simulink model "sampleModel1852"  (R2023a)
settings: Solver=VariableStepAuto  StartTime=0.0  StopTime=10.0  RelTol=1e-3
libraries: hdlsllib x3, simulink x2
settings Model: Creator=user1  LastModifiedBy=user1

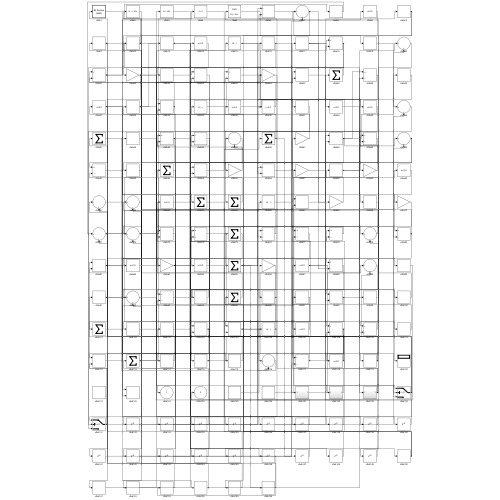
[thumbnail: Simulink's stored preview of the top-level diagram]
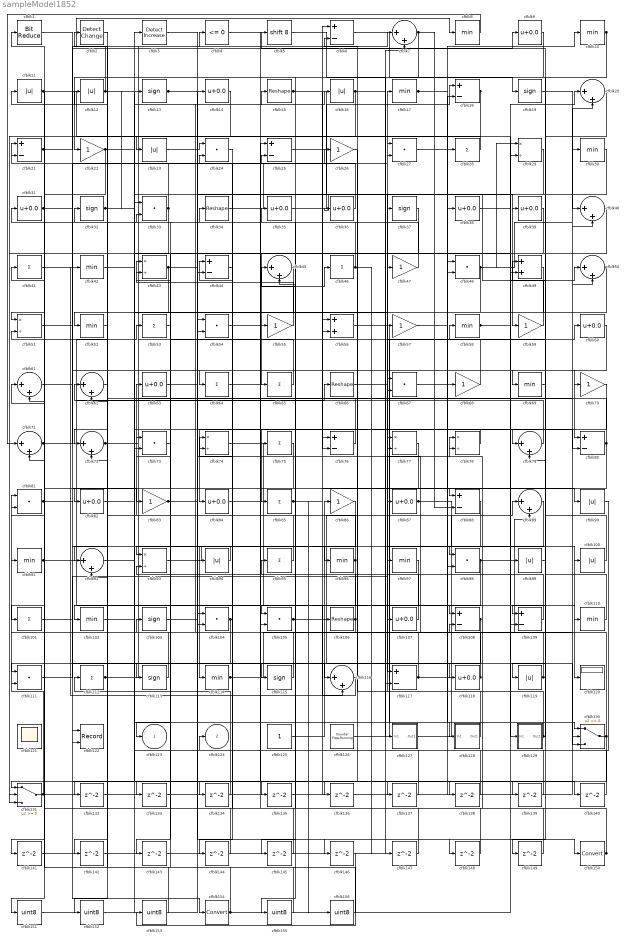
== system sampleModel1852 ==
  cfblk1 : hdlsllib/Logic and Bit Operations/Bit Reduce  mode=AND
  cfblk{8,10,17,30,42,52,58,69,91,96..97,102,110,114} (14 alike) : MinMax
  cfblk{11..12,16,23,90,94,99..100,119} (9 alike) : Abs  SaturateOnIntegerOverflow=off
  cfblk{28,41,46,53,64..65,75,85,95,101,112} (11 alike) : Sum  Inputs=+
  cfblk{13,19,32,37,103,113,115} (7 alike) : Signum
  cfblk{24,27,33,48,54,67,73,81,98,104..105,111} (12 alike) : DotProduct  OutDataTypeStr=Inherit: Inherit via internal rule
  cfblk{15,34,66,106} (4 alike) : Reshape
  cfblk{9,14,31,35..36,38..39,60,63,82,84,87,107,118} (14 alike) : Bias  Bias=0.0  SaturateOnIntegerOverflow=off
  cfblk{6,18,21,25,44,76,80,88,108..109,117} (11 alike) : Sum  Inputs=+-
  cfblk{7,20,40,45,50,61..62,71..72,79,89,92,116} (13 alike) : Sum  Inputs=|++
  cfblk120 : Display
  cfblk121 : Scope
      settings: Floating=on
  cfblk122 : Record  FileSettingsInternal="{\"entries\":[{\"content\":{\"excelSettings\":{\"content\":{},\"type\":\"Streamout.ExcelSettings\"}},\"type\":\"Streamout.FileSettingStorage\",\"uuid\":\"\"}],\"packageUris\":[\"http:\\/\\/schema.mathworks.com\\/mf0\\/streamout_blocks\\/R2020a\"],\"version\":\"1.0\"}"  Layout=[1 1]  SignalsInternal="{\"entries\":[{\"content\":{\"signals\":[{\"content\":{\"blockPath\":[],\"dimensions\":[1],\"domain\":\"\",\"lineColor\":\"#a2142f\",\"plots\":[1],\"port\":1,\"signalID\":4562,\"signalName\":\"XY Graph:1\"},\"type\":\"RecordBlkView.Signal\",\"uuid\":\"\"},{\"content\":{\"blockPath\":[],\"dimensions\":[1],\"domain\":\"\",\"lineColor\":\"#139fff\",\"plots\":[1],\"port\":2,\"signalID\":4565,\"signalName\":\"XY Graph:2\"},\"type\":\"RecordBlkView.Signal\",\"uuid\":\"\"}]},\"type\":\"RecordBlkView.InputSignals\",\"uuid\":\"\"}],\"packageUris\":[\"http:\\/\\/schema.mathworks.com\\/mf0\\/streamout_blocks\\/R2020a\"],\"version\":\"1.0\"}"  VisualizationBindings="{\"xyplotplugin\":{\"info\":[{\"series\":[{\"bindingParametersList\":[{\"parameter\":\"X-Axis\",\"signalID\":4562,\"signalName\":\"XY Graph:1\"},{\"parameter\":\"Y-Axis\",\"signalID\":4565,\"signalName\":\"XY Graph:2\"}],\"seriesID\":56059}],\"subplotID\":1}]}}"  CompatibilityTag=XY  st=-1
  cfblk125 : Constant  SampleTime=-1
  cfblk126 : hdlsllib/Sources/Counter Free-Running  NumBits=16  tsamp=-1
  cfblk127 : Subsystem
      settings: LibrarySourceBlock=|
      | hdlsllib/Ports &
      | Subsystems/Subsystem
  cfblk128 : Subsystem
      settings: LibrarySourceBlock=|
      | hdlsllib/Ports &
      | Subsystems/Subsystem
  cfblk129 : Subsystem
      settings: LibrarySourceBlock=|
      | hdlsllib/Ports &
      | Subsystems/Subsystem
  cfblk130 : Switch  SaturateOnIntegerOverflow=off  InputSameDT=off
  cfblk131 : Switch  SaturateOnIntegerOverflow=off  InputSameDT=off
  cfblk{132..149} (18 alike) : Delay  SampleTime=1
  cfblk150 : DataTypeConversion  SaturateOnIntegerOverflow=off  RndMeth=Floor
  cfblk{151..153,155..156} (5 alike) : DataTypeConversion  OutDataTypeStr=uint8  SaturateOnIntegerOverflow=off  RndMeth=Floor
  cfblk154 : DataTypeConversion  SaturateOnIntegerOverflow=off  RndMeth=Floor
  cfblk2 : simulink/Logic and Bit Operations/Detect Change  vinit=0  OutDataTypeStr=boolean
      settings: LibrarySourceBlock=|
      | hdlsllib/Logic and Bit
      | Operations/Detect
      | Change
  cfblk{22,26,47,55,57,59,68,70,83,86} (10 alike) : Gain
  cfblk{29,43,51,74,77..78,93} (7 alike) : Product  Inputs=*/  RndMeth=Zero  SaturateOnIntegerOverflow=on
  cfblk3 : simulink/Logic and Bit Operations/Detect Increase  vinit=0.0  OutDataTypeStr=boolean
      settings: LibrarySourceBlock=|
      | hdlsllib/Logic and Bit
      | Operations/Detect
      | Increase
  cfblk4 : hdlsllib/Logic and Bit Operations/Compare To Zero  relop=<=  OutDataTypeStr=boolean
  cfblk49 : Sum
  cfblk5 : ArithShift  BitShiftNumber=8
  cfblk56 : Sum
  cfblk123 : Outport  VectorParamsAs1DForOutWhenUnconnected=off
  cfblk124 : Outport  Port=2  VectorParamsAs1DForOutWhenUnconnected=off
  wires:
  cfblk127/1(Out1) -> cfblk89/1
  cfblk74/1 -> cfblk108/1
  cfblk112/1 -> cfblk4/1, cfblk27/2
  cfblk78/1 -> cfblk84/1
  cfblk106/1 -> cfblk15/1, cfblk73/1
  cfblk73/1 -> cfblk112/1
  cfblk116/1 -> cfblk42/1
  cfblk46/1 -> cfblk32/1, cfblk147/1
  cfblk81/1 -> cfblk116/1, cfblk140/1
  cfblk110/1 -> cfblk58/1
  cfblk125/1 -> cfblk86/1
  cfblk113/1 -> cfblk103/1
  cfblk35/1 -> cfblk18/1
  cfblk131/1 -> cfblk81/1, cfblk75/1
  cfblk37/1 -> cfblk65/1
  cfblk28/1 -> cfblk23/1
  cfblk91/1 -> cfblk53/1, cfblk116/2
  cfblk31/1 -> cfblk98/1, cfblk64/1, cfblk51/1
  cfblk59/1 -> cfblk36/1
  cfblk72/1 -> cfblk28/1, cfblk50/2
  cfblk32/1 -> cfblk13/1, cfblk49/2
  cfblk1/1 -> cfblk122/1
  cfblk50/1 -> cfblk105/1, cfblk73/2
  cfblk94/1 -> cfblk93/1
  cfblk87/1 -> cfblk120/1, cfblk90/1
  cfblk96/1 -> cfblk63/1, cfblk145/1
  cfblk33/1 -> cfblk21/1, cfblk131/2
  cfblk15/1 -> cfblk59/1, cfblk37/1
  cfblk22/1 -> cfblk39/1, cfblk71/2, cfblk130/3
  cfblk128/1(Out1) -> cfblk17/1
  cfblk9/1 -> cfblk55/1
  cfblk93/1 -> cfblk100/1
  cfblk3/1 -> cfblk150/1
  cfblk119/1 -> cfblk91/1, cfblk106/1
  cfblk67/1 -> cfblk48/2
  cfblk130/1 -> cfblk81/2, cfblk34/1, cfblk77/2, cfblk141/1
  cfblk107/1 -> cfblk44/1
  cfblk83/1 -> cfblk78/1, cfblk148/1
  cfblk56/1 -> cfblk128/1(In1)
  cfblk117/1 -> cfblk30/1, cfblk21/2
  cfblk102/1 -> cfblk16/1
  cfblk58/1 -> cfblk50/1, cfblk70/1
  cfblk19/1 -> cfblk40/1
  cfblk114/1 -> cfblk89/2, cfblk74/2
  cfblk55/1 -> cfblk43/1
  cfblk40/1 -> cfblk45/2
  cfblk70/1 -> cfblk85/1
  cfblk43/1 -> cfblk52/1, cfblk137/1
  cfblk86/1 -> cfblk114/1
  cfblk90/1 -> cfblk124/1
  cfblk71/1 -> cfblk66/1, cfblk25/2
  cfblk104/1 -> cfblk144/1, cfblk151/1
  cfblk105/1 -> cfblk20/1, cfblk130/2
  cfblk65/1 -> cfblk43/2
  cfblk79/1 -> cfblk62/1
  cfblk47/1 -> cfblk31/1
  cfblk108/1 -> cfblk111/1, cfblk118/1
  cfblk30/1 -> cfblk76/2
  cfblk60/1 -> cfblk80/1
  cfblk53/1 -> cfblk113/1
  cfblk95/1 -> cfblk62/2
  cfblk12/1 -> cfblk8/1, cfblk57/1
  cfblk80/1 -> cfblk101/1, cfblk51/2
  cfblk45/1 -> cfblk102/1
  cfblk27/1 -> cfblk38/1
  cfblk64/1 -> cfblk79/1
  cfblk76/1 -> cfblk11/1
  cfblk84/1 -> cfblk105/2
  cfblk51/1 -> cfblk83/1
  cfblk126/1 -> cfblk60/1
  cfblk20/1 -> cfblk109/1
  cfblk101/1 -> cfblk115/1
  cfblk36/1 -> cfblk1/1
  cfblk6/1 -> cfblk19/1
  cfblk34/1 -> cfblk27/1
  cfblk49/1 -> cfblk123/1
  cfblk118/1 -> cfblk41/1, cfblk12/1
  cfblk18/1 -> cfblk56/2, cfblk131/3
  cfblk115/1 -> cfblk74/1
  cfblk89/1 -> cfblk117/1
  cfblk14/1 -> cfblk72/1
  cfblk25/1 -> cfblk107/1
  cfblk66/1 -> cfblk67/1
  cfblk7/1 -> cfblk22/1, cfblk68/1
  cfblk48/1 -> cfblk20/2, cfblk29/1, cfblk54/2
  cfblk54/1 -> cfblk46/1
  cfblk17/1 -> cfblk10/1, cfblk130/1, cfblk88/2
  cfblk85/1 -> cfblk88/1, cfblk67/2, cfblk156/1
  cfblk23/1 -> cfblk24/1
  cfblk109/1 -> cfblk87/1
  cfblk68/1 -> cfblk47/1
  cfblk38/1 -> cfblk99/1
  cfblk16/1 -> cfblk80/2, cfblk92/2
  cfblk99/1 -> cfblk49/1
  cfblk63/1 -> cfblk104/1
  cfblk10/1 -> cfblk119/1, cfblk92/1
  cfblk129/1(Out1) -> cfblk79/2, cfblk6/2, cfblk78/2
  cfblk82/1 -> cfblk26/1
  cfblk13/1 -> cfblk96/1, cfblk146/1
  cfblk11/1 -> cfblk129/1(In1), cfblk131/1
  cfblk61/1 -> cfblk154/1
  cfblk88/1 -> cfblk98/2
  cfblk5/1 -> cfblk127/1(In1)
  cfblk8/1 -> cfblk71/1
  cfblk29/1 -> cfblk44/2
  cfblk111/1 -> cfblk97/1
  cfblk41/1 -> cfblk69/1
  cfblk52/1 -> cfblk82/1
  cfblk77/1 -> cfblk122/2
  cfblk42/1 -> cfblk77/1
  cfblk24/1 -> cfblk94/1
  cfblk100/1 -> cfblk5/1
  cfblk57/1 -> cfblk110/1
  cfblk21/1 -> cfblk7/1, cfblk9/1
  cfblk98/1 -> cfblk109/2, cfblk142/1
  cfblk62/1 -> cfblk132/1
  cfblk132/1 -> cfblk76/1
  cfblk39/1 -> cfblk133/1
  cfblk133/1 -> cfblk6/1
  cfblk44/1 -> cfblk134/1
  cfblk134/1 -> cfblk72/2
  cfblk103/1 -> cfblk135/1
  cfblk135/1 -> cfblk40/2
  cfblk26/1 -> cfblk136/1
  cfblk136/1 -> cfblk18/2
  cfblk137/1 -> cfblk54/1
  cfblk4/1 -> cfblk138/1
  cfblk138/1 -> cfblk33/1
  cfblk92/1 -> cfblk139/1
  cfblk139/1 -> cfblk56/1
  cfblk140/1 -> cfblk48/1
  cfblk141/1 -> cfblk104/2
  cfblk142/1 -> cfblk7/2
  cfblk75/1 -> cfblk143/1
  cfblk143/1 -> cfblk117/2
  cfblk144/1 -> cfblk111/2
  cfblk145/1 -> cfblk24/2
  cfblk147/1 -> cfblk93/2
  cfblk148/1 -> cfblk45/1
  cfblk69/1 -> cfblk149/1
  cfblk149/1 -> cfblk108/2
  cfblk150/1 -> cfblk25/1, cfblk35/1, cfblk95/1
  cfblk151/1 -> cfblk3/1
  cfblk2/1 -> cfblk152/1
  cfblk152/1 -> cfblk14/1
  cfblk146/1 -> cfblk153/1
  cfblk153/1 -> cfblk2/1
  cfblk154/1 -> cfblk29/2, cfblk33/2
  cfblk97/1 -> cfblk155/1
  cfblk155/1 -> cfblk61/1
  cfblk156/1 -> cfblk61/2

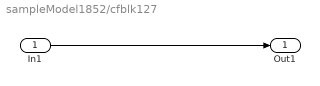
== system sampleModel1852/cfblk127 ==
  In1 : Inport
  Out1 : Outport
  wires:
  In1/1 -> Out1/1

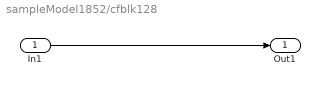
== system sampleModel1852/cfblk128 ==
  In1 : Inport
  Out1 : Outport
  wires:
  In1/1 -> Out1/1

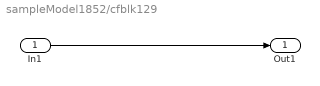
== system sampleModel1852/cfblk129 ==
  In1 : Inport
  Out1 : Outport
  wires:
  In1/1 -> Out1/1
